simulink model "rezervoar13a"  (R2013a)
settings: Solver=ode45  SolverMode=SingleTasking  StartTime=0.0  StopTime=10000.0  RelTol=1e-12  AbsTol=1e-9
undefined symbols (not defined in the file): h0, h10, h20, h30, hmax, q0, s, sout
settings Model: CovMetricSettings=dwe  CovHtmlReporting=off  covSaveCumulativeToWorkspaceVar=off  CovSaveSingleToWorkspaceVar=off  CovExternalEMLEnable=on  Creator=Vukan  LastModifiedBy=Vukan
settings DataIOCC: LimitDataPoints=off  SaveFormat=StructureWithTime
settings DebuggingCC: UnderspecifiedInitializationDetection=Simplified  MergeDetectMultiDrivingBlocksExec=error  SolverPrmCheckMsg=none  FrameProcessingCompatibilityMsg=error  StateNameClashWarn=none  SFUnexpectedBacktrackingDiag=error  SFNoUnconditionalDefaultTransitionDiag=error
settings HardwareCC: ProdBitPerPointer=64  ProdLargestAtomicFloat=Float  ProdIntDivRoundTo=Zero  ProdEndianess=LittleEndian  ProdHWDeviceType=Specified
settings ModelReferenceCC: PropagateSignalLabelsOutOfModel=on
settings GRTTargetCC: CodeReplacementLibrary=C99 (ISO)  GeneratePreprocessorConditionals=Use local settings
settings ConfigurationSet: Description=Simscape Multibody

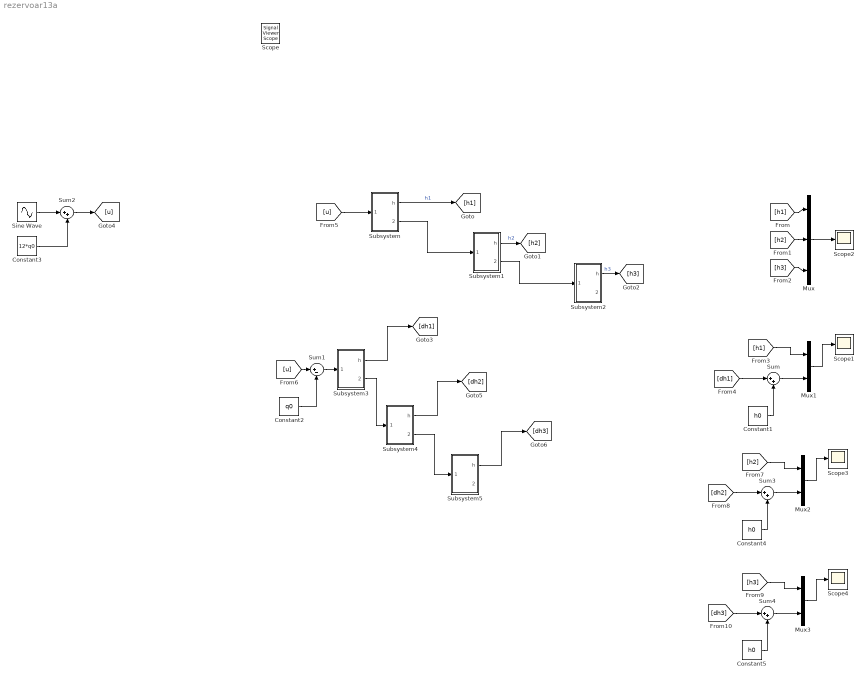
== system rezervoar13a ==
  Constant1 : Constant  Value=h0
  Constant2 : Constant  Value=q0
  Constant3 : Constant  Value=12*q0
  Constant4 : Constant  Value=h0
  Constant5 : Constant  Value=h0
  Mux : Mux  Inputs=3
  Mux1 : Mux  Inputs=2
  Mux2 : Mux  Inputs=2
  Mux3 : Mux  Inputs=2
  Scope{1..4} (4 alike) : Scope
      Scope1 settings: TimeRange=auto  ShowLegends=on  MaxDataPoints=5000  SaveToWorkspace=off  YMin=-5.56932  YMax=80.12391  SampleTime=-1
      Scope2 settings: TimeRange=auto  ShowLegends=on  MaxDataPoints=5000  SaveToWorkspace=off  SaveName=ScopeData2  YMin=2.75  YMax=5.25  SampleTime=-1
      Scope3 settings: TimeRange=auto  ShowLegends=on  MaxDataPoints=5000  SaveToWorkspace=off  SaveName=ScopeData3  YMin=-0.49331  YMax=4.93978  SampleTime=-1
      Scope4 settings: TimeRange=auto  ShowLegends=on  MaxDataPoints=5000  SaveToWorkspace=off  SaveName=ScopeData4  YMin=2.55289  YMax=4.02538  SampleTime=-1
  Sine Wave : Sin  Amplitude=10*q0  Frequency=0.001*30  SampleTime=0
  Subsystem : Subsystem
  Subsystem1 : Subsystem
  Subsystem2 : Subsystem
  Subsystem3 : Subsystem
  Subsystem4 : Subsystem
  Subsystem5 : Subsystem
  Sum{,2..4} (4 alike) : Sum  Inputs=|++
  Sum1 : Sum  Inputs=|+-
  Scope : SignalViewerScope  IOType=viewer  SampleTime=-1  ZoomMode=on
      settings: TimeRange=auto  TickLabels=OneTimeTick  MaxDataPoints=5000  SaveToWorkspace=off  SaveName=ScopeData  YMin=0.00739  YMax=0.01018  SampleInput=off  DataFormat=StructureWithTime
  wires:
  Subsystem/1(h) -> [h1]  "h1"
  Subsystem1/1(h) -> [h2]  "h2"
  Subsystem/2(qout) -> Subsystem1/1(qin)
  Subsystem1/2(qout) -> Subsystem2/1(qin)
  Subsystem2/1(h) -> [h3]  "h3"
  Mux/1 -> Scope2/1
  [h1] -> Mux/1
  [h2] -> Mux/2
  [h3] -> Mux/3
  Subsystem3/1(h) -> [dh1]
  Mux1/1 -> Scope1/1
  [h1] -> Mux1/1
  [dh1] -> Sum/1
  Sum/1 -> Mux1/2
  Constant1/1 -> Sum/2
  [u] -> Subsystem/1(qin)
  [u] -> Sum1/1
  Sum1/1 -> Subsystem3/1(delta qin)
  Constant2/1 -> Sum1/2
  Sine Wave/1 -> Sum2/1
  Sum2/1 -> [u]
  Constant3/1 -> Sum2/2
  Subsystem4/1(h) -> [dh2]
  Subsystem5/1(h) -> [dh3]
  Subsystem3/2(qout) -> Subsystem4/1(delta qin)
  Subsystem4/2(qout) -> Subsystem5/1(delta qin)
  Mux2/1 -> Scope3/1
  [h2] -> Mux2/1
  [dh2] -> Sum3/1
  Sum3/1 -> Mux2/2
  Constant4/1 -> Sum3/2
  Mux3/1 -> Scope4/1
  [h3] -> Mux3/1
  [dh3] -> Sum4/1
  Sum4/1 -> Mux3/2
  Constant5/1 -> Sum4/2

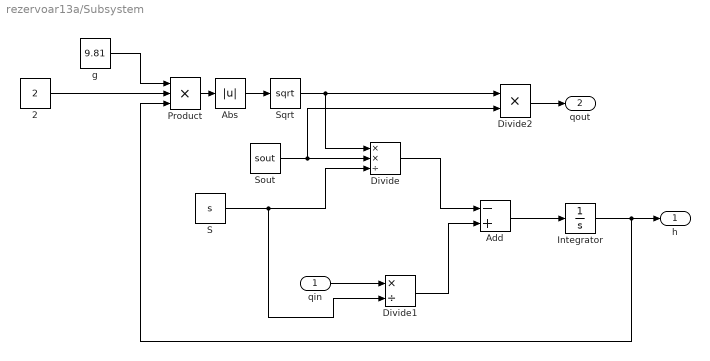
== system rezervoar13a/Subsystem ==
  qin : Inport
  2 : Constant  Value=2
  Abs : Abs
  Add : Sum  Inputs=-+
  Divide : Product  Inputs=**/
  Divide1 : Product  Inputs=*/
  Divide2 : Product  Inputs=**
  Integrator : Integrator  InitialCondition=h10  LimitOutput=on  UpperSaturationLimit=hmax  LowerSaturationLimit=0
  Product : Product  Inputs=3
  "S " : Constant  Value=s
  Sout : Constant  Value=sout
  Sqrt : Sqrt  SaturateOnIntegerOverflow=on
  g : Constant  Value=9.81
  h : Outport
  qout : Outport  Port=2
  wires:
  Sout/1 -> Divide2/2, Divide/2
  "S "/1 -> Divide1/2, Divide/3
  Divide/1 -> Add/1
  qin/1 -> Divide1/1
  Add/1 -> Integrator/1
  g/1 -> Product/1
  Divide1/1 -> Add/2
  Sqrt/1 -> Divide2/1, Divide/1
  2/1 -> Product/2
  Product/1 -> Abs/1
  Abs/1 -> Sqrt/1
  Integrator/1 -> h/1, Product/3
  Divide2/1 -> qout/1

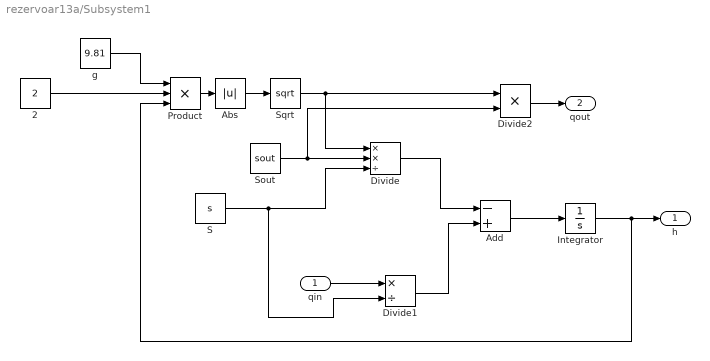
== system rezervoar13a/Subsystem1 ==
  qin : Inport
  2 : Constant  Value=2
  Abs : Abs
  Add : Sum  Inputs=-+
  Divide : Product  Inputs=**/
  Divide1 : Product  Inputs=*/
  Divide2 : Product  Inputs=**
  Integrator : Integrator  InitialCondition=h20  LimitOutput=on  UpperSaturationLimit=hmax  LowerSaturationLimit=0
  Product : Product  Inputs=3
  "S " : Constant  Value=s
  Sout : Constant  Value=sout
  Sqrt : Sqrt  SaturateOnIntegerOverflow=on
  g : Constant  Value=9.81
  h : Outport
  qout : Outport  Port=2
  wires:
  Divide2/1 -> qout/1
  Integrator/1 -> Product/3, h/1
  Abs/1 -> Sqrt/1
  Product/1 -> Abs/1
  2/1 -> Product/2
  Sqrt/1 -> Divide/1, Divide2/1
  Divide1/1 -> Add/2
  g/1 -> Product/1
  Add/1 -> Integrator/1
  qin/1 -> Divide1/1
  Divide/1 -> Add/1
  "S "/1 -> Divide/3, Divide1/2
  Sout/1 -> Divide/2, Divide2/2

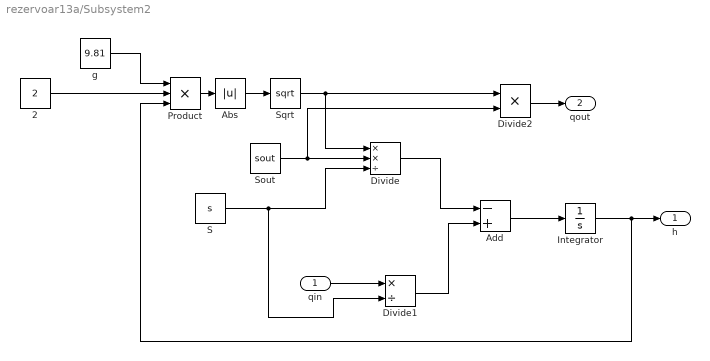
== system rezervoar13a/Subsystem2 ==
  qin : Inport
  2 : Constant  Value=2
  Abs : Abs
  Add : Sum  Inputs=-+
  Divide : Product  Inputs=**/
  Divide1 : Product  Inputs=*/
  Divide2 : Product  Inputs=**
  Integrator : Integrator  InitialCondition=h30  LimitOutput=on  UpperSaturationLimit=hmax  LowerSaturationLimit=0
  Product : Product  Inputs=3
  "S " : Constant  Value=s
  Sout : Constant  Value=sout
  Sqrt : Sqrt  SaturateOnIntegerOverflow=on
  g : Constant  Value=9.81
  h : Outport
  qout : Outport  Port=2
  wires:
  Sout/1 -> Divide2/2, Divide/2
  "S "/1 -> Divide1/2, Divide/3
  Divide/1 -> Add/1
  qin/1 -> Divide1/1
  Add/1 -> Integrator/1
  g/1 -> Product/1
  Divide1/1 -> Add/2
  Sqrt/1 -> Divide2/1, Divide/1
  2/1 -> Product/2
  Product/1 -> Abs/1
  Abs/1 -> Sqrt/1
  Integrator/1 -> h/1, Product/3
  Divide2/1 -> qout/1

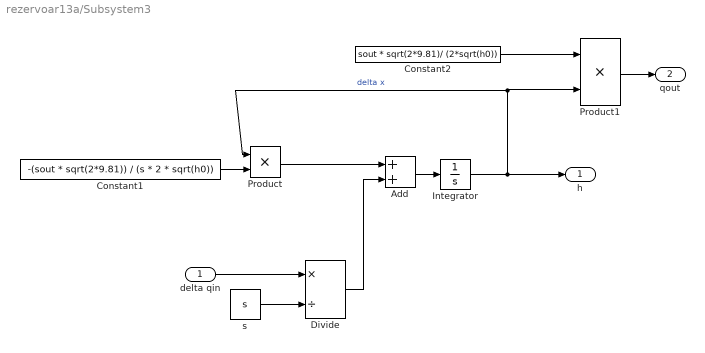
== system rezervoar13a/Subsystem3 ==
  delta qin : Inport
  Add : Sum
  Constant1 : Constant  Value=-(sout * sqrt(2*9.81)) / (s * 2 * sqrt(h0))
  Constant2 : Constant  Value=sout * sqrt(2*9.81)/ (2*sqrt(h0))
  Divide : Product  Inputs=*/
  Integrator : Integrator
  Product : Product
  Product1 : Product
  s : Constant  Value=s
  h : Outport
  qout : Outport  Port=2
  wires:
  Integrator/1 -> h/1, Product1/2, Product/1  "delta x"
  Product/1 -> Add/1
  Add/1 -> Integrator/1
  delta qin/1 -> Divide/1
  Product1/1 -> qout/1
  Divide/1 -> Add/2
  Constant2/1 -> Product1/1
  Constant1/1 -> Product/2
  s/1 -> Divide/2

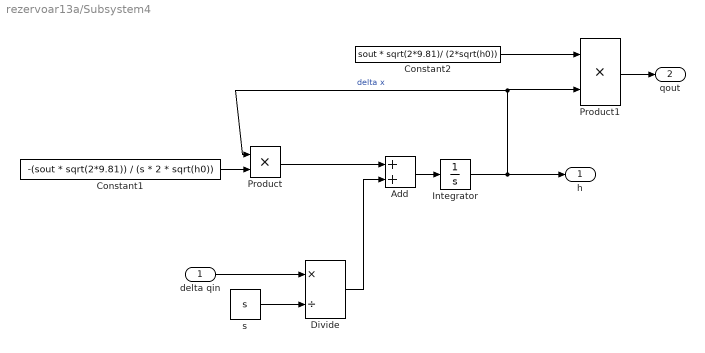
== system rezervoar13a/Subsystem4 ==
  delta qin : Inport
  Add : Sum
  Constant1 : Constant  Value=-(sout * sqrt(2*9.81)) / (s * 2 * sqrt(h0))
  Constant2 : Constant  Value=sout * sqrt(2*9.81)/ (2*sqrt(h0))
  Divide : Product  Inputs=*/
  Integrator : Integrator
  Product : Product
  Product1 : Product
  s : Constant  Value=s
  h : Outport
  qout : Outport  Port=2
  wires:
  s/1 -> Divide/2
  Constant1/1 -> Product/2
  Constant2/1 -> Product1/1
  Divide/1 -> Add/2
  Product1/1 -> qout/1
  delta qin/1 -> Divide/1
  Add/1 -> Integrator/1
  Product/1 -> Add/1
  Integrator/1 -> Product/1, Product1/2, h/1  "delta x"

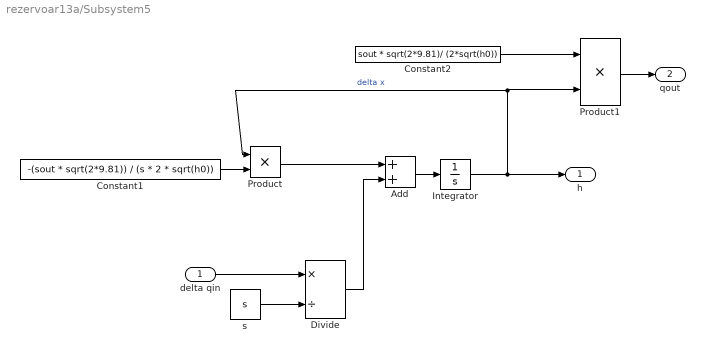
== system rezervoar13a/Subsystem5 ==
  delta qin : Inport
  Add : Sum
  Constant1 : Constant  Value=-(sout * sqrt(2*9.81)) / (s * 2 * sqrt(h0))
  Constant2 : Constant  Value=sout * sqrt(2*9.81)/ (2*sqrt(h0))
  Divide : Product  Inputs=*/
  Integrator : Integrator
  Product : Product
  Product1 : Product
  s : Constant  Value=s
  h : Outport
  qout : Outport  Port=2
  wires:
  Integrator/1 -> h/1, Product1/2, Product/1  "delta x"
  Product/1 -> Add/1
  Add/1 -> Integrator/1
  delta qin/1 -> Divide/1
  Product1/1 -> qout/1
  Divide/1 -> Add/2
  Constant2/1 -> Product1/1
  Constant1/1 -> Product/2
  s/1 -> Divide/2
